simulink model "Controller_Step_12"  (Simulink 7.9)
settings: Solver=FixedStepDiscrete  StartTime=0.0  StopTime=100  FixedStep=0.5  MaxStep=1  RelTol=1e-3
PostLoadFcn:
  | m = 150;
libraries: simulink x3
settings Model: Creator=wcampbel  LastModifiedBy=wcampbel
settings DataIOCC: SaveOutput=off  SaveTime=off
settings OptimizationCC: InlineParams=on  OptimizeModelRefInitCode=on
settings DebuggingCC: FcnCallInpInsideContextMsg=Use local settings  StrictBusMsg=Warning
settings SFSimCC: SimParseCustomCode=off
settings RTWCC: SystemTargetFile=ert.tlc  GenCodeOnly=on  GenerateMakefile=off  TemplateMakefile=ert_default_tmf  Description=Real-Time Workshop Embedded Coder  GenerateReport=on  RTWVerbose=off  ProcessScript=ert_make_rtw_hook  IncludeHyperlinkInReport=on  LaunchReport=on  GenerateTraceInfo=on  GenerateTraceReport=on  GenerateTraceReportSl=on  GenerateTraceReportSf=on  GenerateTraceReportEml=on
settings CodeAppCC: IgnoreCustomStorageClasses=off  SimulinkDataObjDesc=on  SFDataObjDesc=on  CustomSymbolStrGlobalVar=$N$M  CustomSymbolStrBlkIO=$N$M  InsertBlockDesc=on  ReqsInCode=on
settings ERTTargetCC: CodeReplacementLibrary=ANSI_C  MultiwordLength=2048  IncludeMdlTerminateFcn=off  SupportAbsoluteTime=off  SupportNonFinite=off  SupportComplex=off  InlinedParameterPlacement=NonHierarchical  ERTCustomFileTemplate=example_file_process.tlc  ConvertIfToSwitch=off  SuppressUnreachableDefaultCases=off

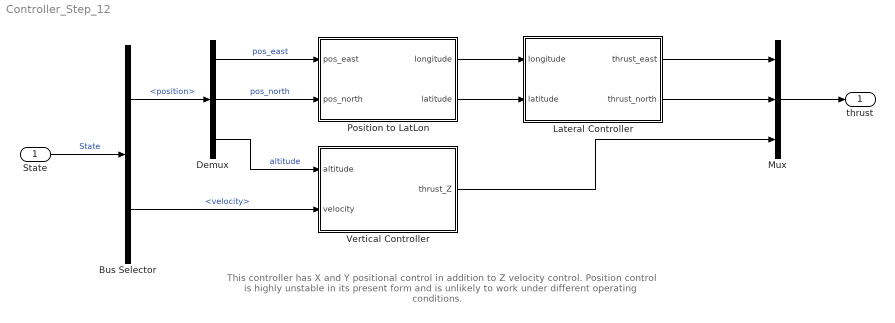
== system Controller_Step_12 ==
  note: This controller has X and Y positional control in addition to Z velocity control.
      | Position control is highly unstable in its present form and is unlikely to work under different operating conditions.
  State : Inport  Description=This variable defines the state of a vehicle under controlled descent. The first element is position in meters. The second is velocity in meters per second.  OutDataTypeStr=Bus: stateBus
  Bus Selector : BusSelector  OutputSignals=position,velocity
  Demux : Demux  Outputs=3
  Lateral Controller : Subsystem
  Mux : Mux  Inputs=3
  Position to LatLon : Subsystem  mask(Position to Latitude and Longitude Conversion){lat0=28.504947, lon0=-80.64105}
      mask prompts: lat0 "Initial Latitude [deg]"; lon0 "Initial Longitude [deg]"
      mask help:
      | This subsystem provides the latitude and longitude of a position on or above the Earth's surface. The user supplies an initial set of coordinates in degrees via the mask. Inputs to the system are the deviation east and north of the coordinate specified in meters.
      |
      | Note that if in the western hemisphere, longitude should be negative.
      mask init:
      | % Define conversion from meters to minutes of longitude based on initial
      | % latitude. Note that the latitude range is limited.
      | 
      | latitude_data     = [30:5:50];
      | meters_per_minute = [1608 1522 1423 1314 1195];
      | 
      | % Find conversion
      | meters_per_lon = interp1(latitude_data,meters_per_minute,lat0,'linear','extrap')*60;
      | 
      | % Define meters per latitude 
      | meters_per_lat = 111118;
  Vertical Controller : Subsystem
  thrust : Outport  OutDataTypeStr=double  PortDimensions=3
  wires:
  Demux/3 -> Vertical Controller/1(altitude)  "altitude"
  Bus Selector/2 -> Vertical Controller/2(velocity)  "<velocity>"
  Bus Selector/1 -> Demux/1  "<position>"
  State/1 -> Bus Selector/1  "State"
  Mux/1 -> thrust/1
  Demux/1 -> Position to LatLon/1(pos_east)  "pos_east"
  Demux/2 -> Position to LatLon/2(pos_north)  "pos_north"
  Position to LatLon/1(longitude) -> Lateral Controller/1(longitude)
  Position to LatLon/2(latitude) -> Lateral Controller/2(latitude)
  Lateral Controller/1(thrust_east) -> Mux/1
  Lateral Controller/2(thrust_north) -> Mux/2
  Vertical Controller/1(thrust_Z) -> Mux/3

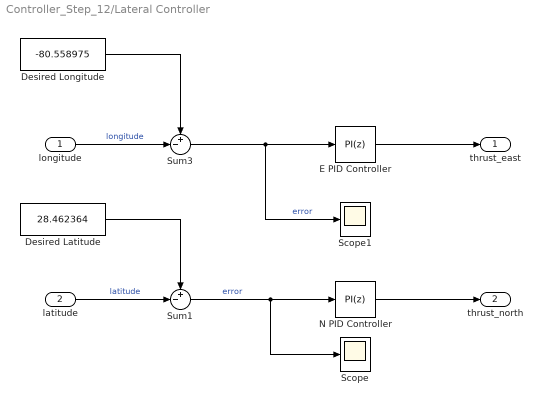
== system Controller_Step_12/Lateral Controller ==
  longitude : Inport
  latitude : Inport  Port=2
  Desired Latitude : Constant  Value=28.462364
  Desired Longitude : Constant  Value=-80.558975
  E PID Controller : simulink/Continuous/PID Controller  Controller=PI  TimeDomain=Discrete-time  SampleTime=0.5  IntegratorMethod=Forward Euler  FilterMethod=Forward Euler  Form=Parallel  P=260000  I=0  D=0  N=100  InitialConditionSource=internal  InitialConditionForIntegrator=0  InitialConditionForFilter=0  ExternalReset=none  ZeroCross=off  LimitOutput=off  UpperSaturationLimit=inf  LowerSaturationLimit=0  LinearizeAsGain=off  AntiWindupMode=none  Kb=1  TrackingMode=off  Kt=1  PParamMin=[]  PParamMax=[]  IParamMin=[]  IParamMax=[]  DParamMin=[]  DParamMax=[]  NParamMin=[]  NParamMax=[]  KbParamMin=[]  KbParamMax=[]  KtParamMin=[]  KtParamMax=[]  POutMin=[]  POutMax=[]  IOutMin=[]  IOutMax=[]  DOutMin=[]  DOutMax=[]  NOutMin=[]  NOutMax=[]  KbOutMin=[]  KbOutMax=[]  KtOutMin=[]  KtOutMax=[]  IntegratorOutMin=[]  IntegratorOutMax=[]  FilterOutMin=[]  FilterOutMax=[]  SumOutMin=[]  SumOutMax=[]  SumI1OutMin=[]  SumI1OutMax=[]  SumI2OutMin=[]  SumI2OutMax=[]  SumI3OutMin=[]  SumI3OutMax=[]  SumDOutMin=[]  SumDOutMax=[]  SaturationOutMin=[]  SaturationOutMax=[]  IntegratorContinuousStateAttributes=''  IntegratorStateMustResolveToSignalObject=off  IntegratorRTWStateStorageClass=Auto  FilterContinuousStateAttributes=''  FilterStateMustResolveToSignalObject=off  FilterRTWStateStorageClass=Auto
  N PID Controller : simulink/Continuous/PID Controller  Controller=PI  TimeDomain=Discrete-time  SampleTime=0.5  IntegratorMethod=Forward Euler  FilterMethod=Forward Euler  Form=Parallel  P=600000  I=500  D=.1  N=100  InitialConditionSource=internal  InitialConditionForIntegrator=0  InitialConditionForFilter=0  ExternalReset=none  ZeroCross=off  LimitOutput=off  UpperSaturationLimit=inf  LowerSaturationLimit=0  LinearizeAsGain=off  AntiWindupMode=none  Kb=1  TrackingMode=off  Kt=1  PParamMin=[]  PParamMax=[]  IParamMin=[]  IParamMax=[]  DParamMin=[]  DParamMax=[]  NParamMin=[]  NParamMax=[]  KbParamMin=[]  KbParamMax=[]  KtParamMin=[]  KtParamMax=[]  POutMin=[]  POutMax=[]  IOutMin=[]  IOutMax=[]  DOutMin=[]  DOutMax=[]  NOutMin=[]  NOutMax=[]  KbOutMin=[]  KbOutMax=[]  KtOutMin=[]  KtOutMax=[]  IntegratorOutMin=[]  IntegratorOutMax=[]  FilterOutMin=[]  FilterOutMax=[]  SumOutMin=[]  SumOutMax=[]  SumI1OutMin=[]  SumI1OutMax=[]  SumI2OutMin=[]  SumI2OutMax=[]  SumI3OutMin=[]  SumI3OutMax=[]  SumDOutMin=[]  SumDOutMax=[]  SaturationOutMin=[]  SaturationOutMax=[]  IntegratorContinuousStateAttributes=''  IntegratorStateMustResolveToSignalObject=off  IntegratorRTWStateStorageClass=Auto  FilterContinuousStateAttributes=''  FilterStateMustResolveToSignalObject=off  FilterRTWStateStorageClass=Auto
  Scope : Scope
      settings: TimeRange=27.56653992395438  YMin=-2.28914e+007  YMax=-2.07112e+007
  Scope1 : Scope
      settings: TimeRange=27.56653992395438  YMin=0.002072  YMax=0.002086  SaveName=ScopeData2
  Sum1 : Sum  Inputs=+-|
  Sum3 : Sum  Inputs=+-|
  thrust_east : Outport
  thrust_north : Outport  Port=2
  wires:
  E PID Controller/1 -> thrust_east/1
  Sum3/1 -> E PID Controller/1, Scope1/1  "error"
  longitude/1 -> Sum3/2  "longitude"
  Desired Longitude/1 -> Sum3/1
  Desired Latitude/1 -> Sum1/1
  latitude/1 -> Sum1/2  "latitude"
  Sum1/1 -> N PID Controller/1, Scope/1  "error"
  N PID Controller/1 -> thrust_north/1

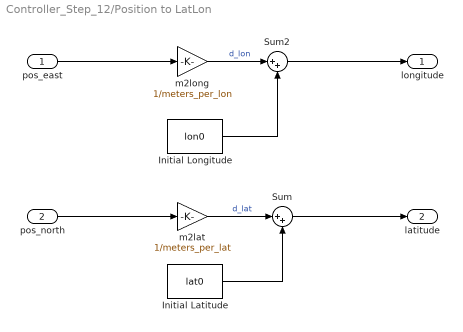
== system Controller_Step_12/Position to LatLon ==
  pos_east : Inport
  pos_north : Inport  Port=2
  Initial Latitude : Constant  Value=lat0
  Initial Longitude : Constant  Value=lon0
  Sum : Sum  Inputs=|++
  Sum2 : Sum  Inputs=|++
  m2lat : Gain  Gain=1/meters_per_lat
  m2long : Gain  Gain=1/meters_per_lon
  longitude : Outport
  latitude : Outport  Port=2
  wires:
  m2lat/1 -> Sum/1  "d_lat"
  Initial Latitude/1 -> Sum/2
  m2long/1 -> Sum2/1  "d_lon"
  Initial Longitude/1 -> Sum2/2
  pos_north/1 -> m2lat/1
  pos_east/1 -> m2long/1
  Sum2/1 -> longitude/1
  Sum/1 -> latitude/1

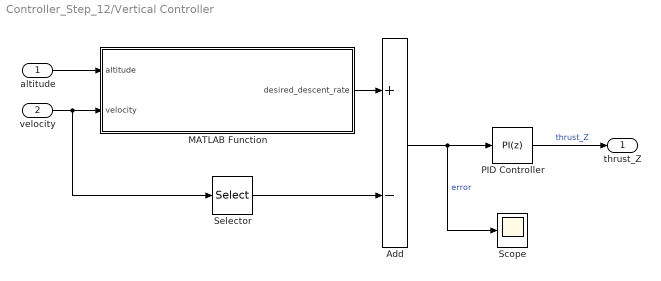
== system Controller_Step_12/Vertical Controller ==
  altitude : Inport
  velocity : Inport  Port=2
  Add : Sum  Inputs=+-
  MATLAB Function : MATLAB Function  TreatAsAtomicUnit=on
  PID Controller : simulink/Continuous/PID Controller  Controller=PI  TimeDomain=Discrete-time  SampleTime=0.5  IntegratorMethod=Forward Euler  FilterMethod=Forward Euler  Form=Parallel  P=50  I=5  D=0  N=100  InitialConditionSource=internal  InitialConditionForIntegrator=0  InitialConditionForFilter=0  ExternalReset=none  LimitOutput=on  UpperSaturationLimit=inf  LowerSaturationLimit=0  LinearizeAsGain=off  AntiWindupMode=none  Kb=1  TrackingMode=off  Kt=1  PParamMin=[]  PParamMax=[]  IParamMin=[]  IParamMax=[]  DParamMin=[]  DParamMax=[]  NParamMin=[]  NParamMax=[]  KbParamMin=[]  KbParamMax=[]  KtParamMin=[]  KtParamMax=[]  POutMin=[]  POutMax=[]  IOutMin=[]  IOutMax=[]  DOutMin=[]  DOutMax=[]  NOutMin=[]  NOutMax=[]  KbOutMin=[]  KbOutMax=[]  KtOutMin=[]  KtOutMax=[]  IntegratorOutMin=[]  IntegratorOutMax=[]  FilterOutMin=[]  FilterOutMax=[]  SumOutMin=[]  SumOutMax=[]  SumI1OutMin=[]  SumI1OutMax=[]  SumI2OutMin=[]  SumI2OutMax=[]  SumI3OutMin=[]  SumI3OutMax=[]  SumDOutMin=[]  SumDOutMax=[]  SaturationOutMin=[]  SaturationOutMax=[]  IntegratorContinuousStateAttributes=''  IntegratorStateMustResolveToSignalObject=off  IntegratorRTWStateStorageClass=Auto  FilterContinuousStateAttributes=''  FilterStateMustResolveToSignalObject=off  FilterRTWStateStorageClass=Auto
  Scope : Scope
      settings: ShowLegends=on  TimeRange=27.56653992395438  YMin=-10  YMax=19.90625
  Selector : Selector  InputPortWidth=3  IndexOptions=Index vector (dialog)  Indices=3  OutputSizes=1
  thrust_Z : Outport
  wires:
  MATLAB Function/1(desired_descent_rate) -> Add/1
  Add/1 -> PID Controller/1, Scope/1  "error"
  velocity/1 -> MATLAB Function/2(velocity), Selector/1
  altitude/1 -> MATLAB Function/1(altitude)
  PID Controller/1 -> thrust_Z/1  "thrust_Z"
  Selector/1 -> Add/2

== matlab function Vertical Controller/MATLAB Function ==
  data: altitude input double; desired_descent_rate output double; velocity input double
function desired_descent_rate = variable_v(altitude,velocity)

height = altitude - 5;

if height > 500
   desired_descent_rate = velocity(3);
elseif height > 200
   desired_descent_rate = -10;
elseif height > 100
   desired_descent_rate = -2;
elseif height > 10
   desired_descent_rate = -1;
else
   desired_descent_rate = -0.5;
end
